simulink model "Appl_PaLearn_CtrlModel"  (R2018b)
settings: configuration reference "CodeConfig_10_ms" (kept outside this file)
undefined symbols (not defined in the file): CAL_LearnAllTimeMax_150s, CAL_LearnSingleTimeMax_60s, D_FirstMove, D_FourthlyMove, D_Invalid, D_SecondMove, D_ThirdlyMove, enDrAdjustEnable, FALSE, TRUE
libraries: DareLib x52, simulink x2
(part 1 of 2)
settings Model: Creator=Administrator  LastModifiedBy=Administrator
settings ConfigSetRef: SourceLocation=Base Workspace

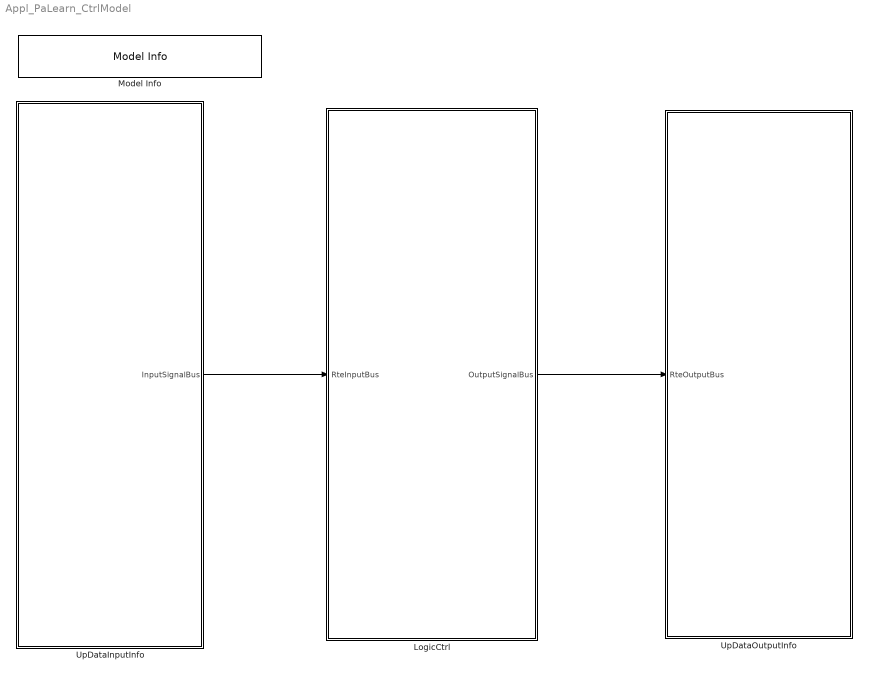
== system Appl_PaLearn_CtrlModel ==
  LogicCtrl : Subsystem  Priority=2  TreatAsAtomicUnit=on
      settings: RTWSystemCode=Nonreusable function  RTWFcnNameOpts=Use subsystem name
  Model Info : simulink/Model-Wide Utilities/Model Info  Frame=on  DisplayStringWithTags=Version：%<ModelVersion>  HorizontalTextAlignment=Center  LeftAlignmentValue=0.5
  UpDataInputInfo : Subsystem  Priority=1  TreatAsAtomicUnit=on
      settings: RTWSystemCode=Nonreusable function  RTWFcnNameOpts=Use subsystem name
  UpDataOutputInfo : Subsystem  Priority=3  TreatAsAtomicUnit=on
      settings: RTWSystemCode=Nonreusable function  RTWFcnNameOpts=Use subsystem name
  wires:
  LogicCtrl/1(OutputSignalBus) -> UpDataOutputInfo/1(RteOutputBus)
  UpDataInputInfo/1(InputSignalBus) -> LogicCtrl/1(RteInputBus)

== system Appl_PaLearn_CtrlModel/LogicCtrl ==
  RteInputBus : Inport
  LocalAdjustCtrl : Subsystem  Description=学习逻辑处理
      settings: AttributesFormatString=%<Description>
  OutputSignalBus : Outport
  wires:
  RteInputBus/1 -> LocalAdjustCtrl/1(RteInputBus)  "RteInputBus"
  LocalAdjustCtrl/1(OutputSignalBus) -> OutputSignalBus/1

== system Appl_PaLearn_CtrlModel/UpDataInputInfo ==
  InputSignalProcess : Subsystem  Description=数据处理
      settings: AttributesFormatString=%<Description>  RTWSystemCode=Nonreusable function  RTWFcnNameOpts=Use subsystem name
  RTE : Subsystem  Description=接口自动生成  TreatAsAtomicUnit=on
      settings: AttributesFormatString=%<Description>  RTWSystemCode=Nonreusable function  RTWFcnNameOpts=Use subsystem name
  InputSignalBus : Outport
  wires:
  InputSignalProcess/1(InputSignalBus) -> InputSignalBus/1
  RTE/1(RTE_Signal) -> InputSignalProcess/1(Rte_SignalBus)

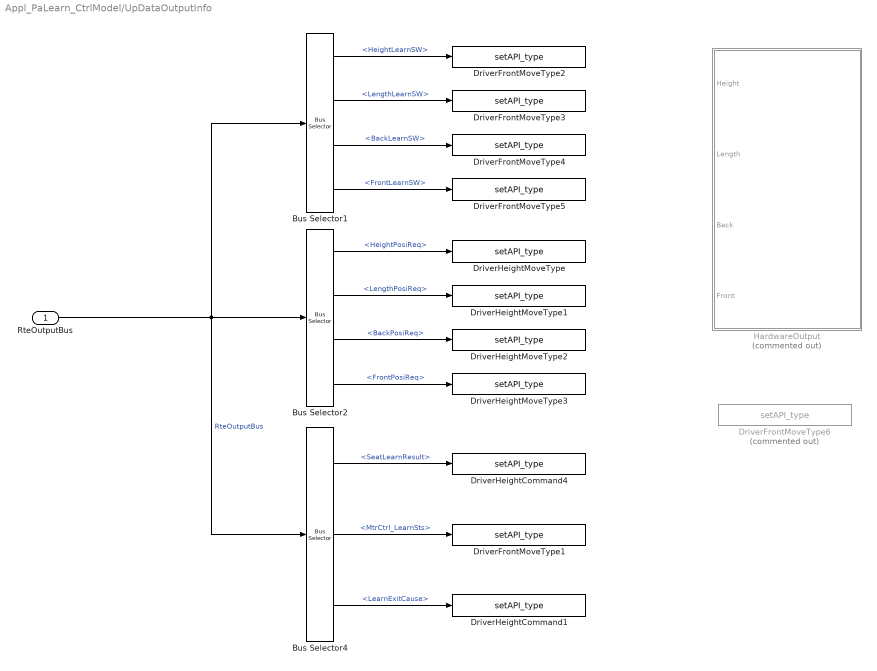
== system Appl_PaLearn_CtrlModel/UpDataOutputInfo ==
  RteOutputBus : Inport
  Bus Selector1 : BusSelector  OutputSignals=LearnOut.HeightLearnSW,LearnOut.LengthLearnSW,LearnOut.BackLearnSW,LearnOut.FrontLearnSW
  Bus Selector2 : BusSelector  OutputSignals=ResetOutBus.HeightPosiReq,ResetOutBus.LengthPosiReq,ResetOutBus.BackPosiReq,ResetOutBus.FrontPosiReq
  Bus Selector4 : BusSelector  OutputSignals=SeatLearnResult,LearnOut.MtrCtrl_LearnSts,LearnOut.LearnExitCause
  DriverFrontMoveType1 : DareLib/Dare/setAPI_type  g_funcname=Rte_SetVfb_PaLearnSts  g_param=""  g_type=uint8  g_enum=enLearnSts  g_size=-1
      settings: AttributesFormatString=%<g_funcname>  SourceProductName=Dare Library
  DriverFrontMoveType2 : DareLib/Dare/setAPI_type  g_funcname=Rte_SetVfb_PaHeightLearnCmd  g_param=""  g_type=uint8  g_enum=enSWMoveCmd  g_size=-1
      settings: AttributesFormatString=%<g_funcname>  SourceProductName=Dare Library
  DriverFrontMoveType3 : DareLib/Dare/setAPI_type  g_funcname=Rte_SetVfb_PaLengthLearnCmd  g_param=""  g_type=uint8  g_enum=enSWMoveCmd  g_size=-1
      settings: AttributesFormatString=%<g_funcname>  SourceProductName=Dare Library
  DriverFrontMoveType4 : DareLib/Dare/setAPI_type  g_funcname=Rte_SetVfb_PaBackLearnCmd  g_param=""  g_type=uint8  g_enum=enSWMoveCmd  g_size=-1
      settings: AttributesFormatString=%<g_funcname>  SourceProductName=Dare Library
  DriverFrontMoveType5 : DareLib/Dare/setAPI_type  g_funcname=Rte_SetVfb_PaFrontLearnCmd  g_param=""  g_type=uint8  g_enum=enSWMoveCmd  g_size=-1
      settings: AttributesFormatString=%<g_funcname>  SourceProductName=Dare Library
  DriverFrontMoveType6 : DareLib/Dare/setAPI_type  Commented=on  g_funcname=Rte_SetVfb_DrLearnResult  g_param=""  g_type=uint8  g_enum=enSeatAutoRunSts  g_size=-1
      settings: AttributesFormatString=%<g_funcname>  SourceProductName=Dare Library
  DriverHeightCommand1 : DareLib/Dare/setAPI_type  g_funcname=Rte_SetVfb_PaLearnExitCause  g_param=""  g_type=uint8  g_enum=enLearnExitCause  g_size=-1
      settings: AttributesFormatString=%<g_funcname>  SourceProductName=Dare Library
  DriverHeightCommand4 : DareLib/Dare/setAPI_type  g_funcname=Rte_SetVfb_PaLearnResult  g_param=""  g_type=uint8  g_size=-1
      settings: AttributesFormatString=%<g_funcname>  SourceProductName=Dare Library
  DriverHeightMoveType : DareLib/Dare/setAPI_type  g_funcname=Rte_SetVfb_PaHeightResetReqPosi  g_param=""  g_type=uint16  g_size=-1
      settings: AttributesFormatString=%<g_funcname>  SourceProductName=Dare Library
  DriverHeightMoveType1 : DareLib/Dare/setAPI_type  g_funcname=Rte_SetVfb_PaLengthResetReqPosi  g_param=""  g_type=uint16  g_size=-1
      settings: AttributesFormatString=%<g_funcname>  SourceProductName=Dare Library
  DriverHeightMoveType2 : DareLib/Dare/setAPI_type  g_funcname=Rte_SetVfb_PaBackResetReqPosi  g_param=""  g_type=uint16  g_size=-1
      settings: AttributesFormatString=%<g_funcname>  SourceProductName=Dare Library
  DriverHeightMoveType3 : DareLib/Dare/setAPI_type  g_funcname=Rte_SetVfb_PaFrontResetReqPosi  g_param=""  g_type=uint16  g_size=-1
      settings: AttributesFormatString=%<g_funcname>  SourceProductName=Dare Library
  HardwareOutput : Subsystem  Commented=on
  wires:
  RteOutputBus/1 -> Bus Selector4/1, Bus Selector1/1, Bus Selector2/1  "RteOutputBus"
  Bus Selector2/4 -> DriverHeightMoveType3/1  "<FrontPosiReq>"
  Bus Selector2/3 -> DriverHeightMoveType2/1  "<BackPosiReq>"
  Bus Selector2/2 -> DriverHeightMoveType1/1  "<LengthPosiReq>"
  Bus Selector2/1 -> DriverHeightMoveType/1  "<HeightPosiReq>"
  Bus Selector4/2 -> DriverFrontMoveType1/1  "<MtrCtrl_LearnSts>"
  Bus Selector4/1 -> DriverHeightCommand4/1  "<SeatLearnResult>"
  Bus Selector1/1 -> DriverFrontMoveType2/1  "<HeightLearnSW>"
  Bus Selector1/2 -> DriverFrontMoveType3/1  "<LengthLearnSW>"
  Bus Selector1/3 -> DriverFrontMoveType4/1  "<BackLearnSW>"
  Bus Selector1/4 -> DriverFrontMoveType5/1  "<FrontLearnSW>"
  Bus Selector4/3 -> DriverHeightCommand1/1  "<LearnExitCause>"

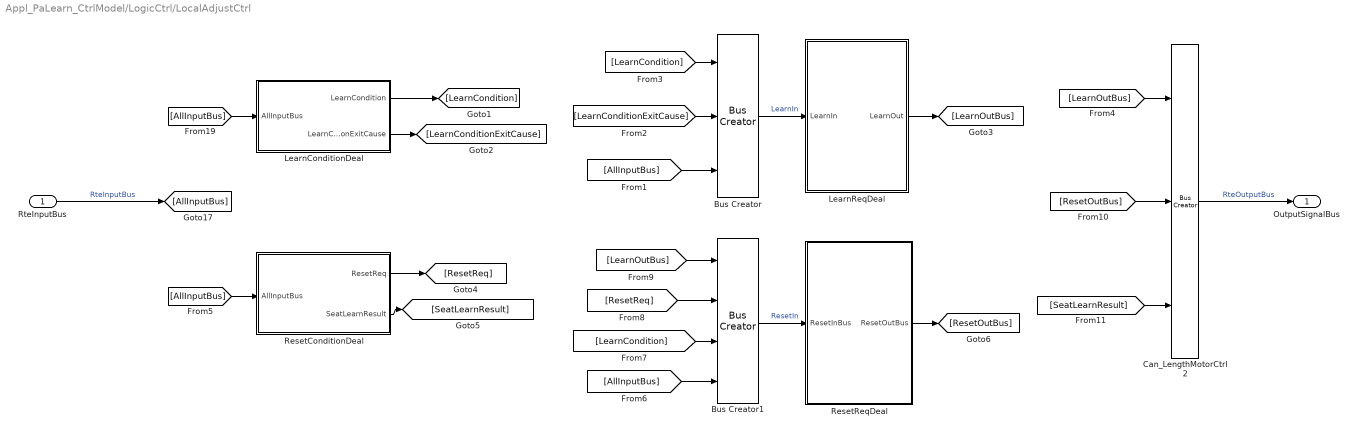
== system Appl_PaLearn_CtrlModel/LogicCtrl/LocalAdjustCtrl ==
  RteInputBus : Inport
  Bus Creator : BusCreator  Inputs=3
  Bus Creator1 : BusCreator  Inputs=4
  Can_LengthMotorCtrl2 : BusCreator  Inputs=3
  LearnConditionDeal : Subsystem
  LearnReqDeal : Subsystem
  ResetConditionDeal : Subsystem
  ResetReqDeal : Subsystem
  OutputSignalBus : Outport
  wires:
  RteInputBus/1 -> [AllInputBus]  "RteInputBus"
  [AllInputBus] -> Bus Creator/3
  [AllInputBus] -> LearnConditionDeal/1(AllInputBus)
  LearnConditionDeal/1(LearnCondition) -> [LearnCondition]
  LearnConditionDeal/2(LearnConditionExitCause) -> [LearnConditionExitCause]
  Bus Creator/1 -> LearnReqDeal/1(LearnIn)  "LearnIn"
  LearnReqDeal/1(LearnOut) -> [LearnOutBus]
  [LearnCondition] -> Bus Creator/1
  [LearnConditionExitCause] -> Bus Creator/2
  [LearnOutBus] -> Can_LengthMotorCtrl2/1
  Can_LengthMotorCtrl2/1 -> OutputSignalBus/1  "RteOutputBus"
  [LearnCondition] -> Bus Creator1/3
  [AllInputBus] -> Bus Creator1/4
  [ResetReq] -> Bus Creator1/2
  Bus Creator1/1 -> ResetReqDeal/1(ResetInBus)  "ResetIn"
  [LearnOutBus] -> Bus Creator1/1
  ResetReqDeal/1(ResetOutBus) -> [ResetOutBus]
  [ResetOutBus] -> Can_LengthMotorCtrl2/2
  [AllInputBus] -> ResetConditionDeal/1(AllInputBus)
  ResetConditionDeal/1(ResetReq) -> [ResetReq]
  ResetConditionDeal/2(SeatLearnResult) -> [SeatLearnResult]
  [SeatLearnResult] -> Can_LengthMotorCtrl2/3

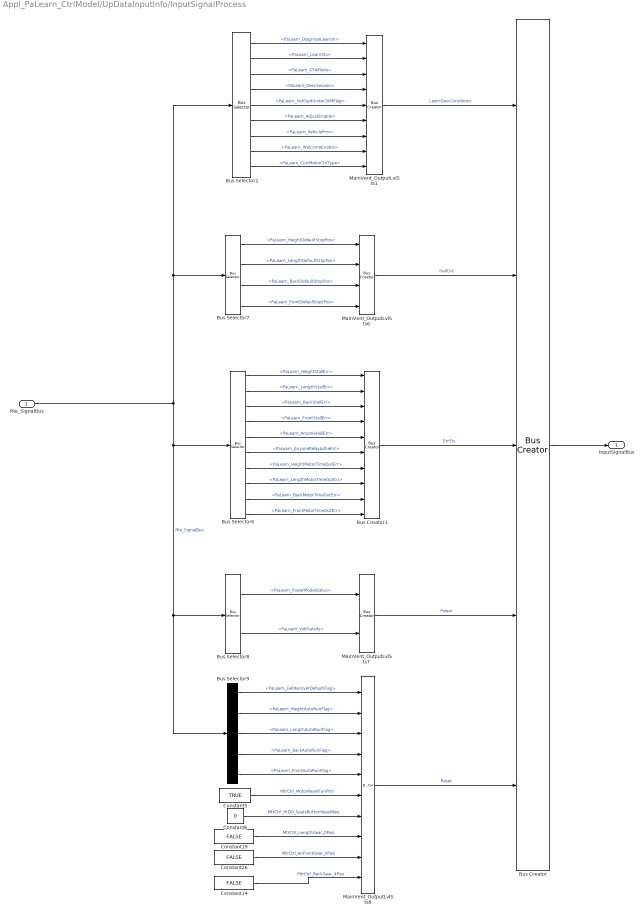
== system Appl_PaLearn_CtrlModel/UpDataInputInfo/InputSignalProcess ==
  Rte_SignalBus : Inport
  Bus Creator : BusCreator  Inputs=5
  Bus Creator1 : BusCreator  Inputs=10
  Bus Selector2 : BusSelector  OutputSignals=PaLearn_DiagnoseLearnIn,PaLearn_LearnSts,PaLearn_OTAMode,PaLearn_DescSession,PaLearn_VehSpdUnder3KMFlag,PaLearn_AdjustEnable,PaLearn_VehiclePrm,PaLearn_WelcomeEnable,PaLearn_CurrMotorCtrlType
  Bus Selector6 : BusSelector  OutputSignals=PaLearn_HeightStallErr,PaLearn_LengthStallErr,PaLearn_BackStallErr,PaLearn_FrontStallErr,PaLearn_AnyoneHallErr,PaLearn_AnyoneRelayAdheErr,PaLearn_HeightMotorTimeOutErr,PaLearn_LengthMotorTimeOutErr,PaLearn_BackMotorTimeOutErr,PaLearn_FrontMotorTimeOutErr
  Bus Selector7 : BusSelector  OutputSignals=PaLearn_HeightDefaultStopPos,PaLearn_LengthDefaultStopPos,PaLearn_BackDefaultStopPos,PaLearn_FrontDefaulStoptPos
  Bus Selector8 : BusSelector  OutputSignals=PaLearn_PowerModeStatus,PaLearn_VoltSatisfy
  Bus Selector9 : BusSelector  OutputSignals=PaLearn_GetRecoverDefaultFlag,PaLearn_HeightAutoRunFlag,PaLearn_LengthAutoRunFlag,PaLearn_BackAutoRunFlag,PaLearn_FrontAutoRunFlag
  Constant14 : Constant  Value=FALSE
  Constant19 : Constant  Value=FALSE
  Constant26 : Constant  Value=FALSE
  Constant5 : Constant  Value=TRUE
  Constant6 : Constant  Value=0
  MainVent_OutputLvlSts1 : BusCreator  Inputs=9
  MainVent_OutputLvlSts6 : BusCreator  Inputs=4
  MainVent_OutputLvlSts7 : BusCreator  Inputs=2
  MainVent_OutputLvlSts8 : BusCreator  Inputs=10
  InputSignalBus : Outport
  wires:
  Bus Creator/1 -> InputSignalBus/1
  Rte_SignalBus/1 -> Bus Selector2/1, Bus Selector7/1, Bus Selector9/1, Bus Selector8/1, Bus Selector6/1  "Rte_SignalBus"
  MainVent_OutputLvlSts7/1 -> Bus Creator/4  "Power"
  Bus Creator1/1 -> Bus Creator/3  "ErrSts"
  MainVent_OutputLvlSts1/1 -> Bus Creator/1  "LearnDescConditions"
  MainVent_OutputLvlSts6/1 -> Bus Creator/2  "HallCnt"
  MainVent_OutputLvlSts8/1 -> Bus Creator/5  "Reset"
  Bus Selector9/1 -> MainVent_OutputLvlSts8/1  "<PaLearn_GetRecoverDefaultFlag>"
  Bus Selector9/2 -> MainVent_OutputLvlSts8/2  "<PaLearn_HeightAutoRunFlag>"
  Bus Selector9/3 -> MainVent_OutputLvlSts8/3  "<PaLearn_LengthAutoRunFlag>"
  Bus Selector9/4 -> MainVent_OutputLvlSts8/4  "<PaLearn_BackAutoRunFlag>"
  Bus Selector9/5 -> MainVent_OutputLvlSts8/5  "<PaLearn_FrontAutoRunFlag>"
  Constant19/1 -> MainVent_OutputLvlSts8/8  "MtrCtrl_LengthGear_0Posi"
  Constant5/1 -> MainVent_OutputLvlSts8/6  "MtrCtrl_MotorResetFunPrm"
  Constant6/1 -> MainVent_OutputLvlSts8/7  "MtrCtrl_HIDO_SeatsButtonResetReq"
  Constant26/1 -> MainVent_OutputLvlSts8/9  "MtrCtrl_enFrontGear_0Posi"
  Constant14/1 -> MainVent_OutputLvlSts8/10  "MtrCtrl_BackGear_4Posi"
  Bus Selector7/3 -> MainVent_OutputLvlSts6/3  "<PaLearn_BackDefaultStopPos>"
  Bus Selector7/2 -> MainVent_OutputLvlSts6/2  "<PaLearn_LengthDefaultStopPos>"
  Bus Selector7/4 -> MainVent_OutputLvlSts6/4  "<PaLearn_FrontDefaulStoptPos>"
  Bus Selector7/1 -> MainVent_OutputLvlSts6/1  "<PaLearn_HeightDefaultStopPos>"
  Bus Selector6/1 -> Bus Creator1/1  "<PaLearn_HeightStallErr>"
  Bus Selector6/2 -> Bus Creator1/2  "<PaLearn_LengthStallErr>"
  Bus Selector6/3 -> Bus Creator1/3  "<PaLearn_BackStallErr>"
  Bus Selector6/4 -> Bus Creator1/4  "<PaLearn_FrontStallErr>"
  Bus Selector6/5 -> Bus Creator1/5  "<PaLearn_AnyoneHallErr>"
  Bus Selector6/6 -> Bus Creator1/6  "<PaLearn_AnyoneRelayAdheErr>"
  Bus Selector6/7 -> Bus Creator1/7  "<PaLearn_HeightMotorTimeOutErr>"
  Bus Selector6/8 -> Bus Creator1/8  "<PaLearn_LengthMotorTimeOutErr>"
  Bus Selector6/9 -> Bus Creator1/9  "<PaLearn_BackMotorTimeOutErr>"
  Bus Selector6/10 -> Bus Creator1/10  "<PaLearn_FrontMotorTimeOutErr>"
  Bus Selector8/2 -> MainVent_OutputLvlSts7/2  "<PaLearn_VoltSatisfy>"
  Bus Selector8/1 -> MainVent_OutputLvlSts7/1  "<PaLearn_PowerModeStatus>"
  Bus Selector2/1 -> MainVent_OutputLvlSts1/1  "<PaLearn_DiagnoseLearnIn>"
  Bus Selector2/2 -> MainVent_OutputLvlSts1/2  "<PaLearn_LearnSts>"
  Bus Selector2/3 -> MainVent_OutputLvlSts1/3  "<PaLearn_OTAMode>"
  Bus Selector2/4 -> MainVent_OutputLvlSts1/4  "<PaLearn_DescSession>"
  Bus Selector2/5 -> MainVent_OutputLvlSts1/5  "<PaLearn_VehSpdUnder3KMFlag>"
  Bus Selector2/6 -> MainVent_OutputLvlSts1/6  "<PaLearn_AdjustEnable>"
  Bus Selector2/7 -> MainVent_OutputLvlSts1/7  "<PaLearn_VehiclePrm>"
  Bus Selector2/8 -> MainVent_OutputLvlSts1/8  "<PaLearn_WelcomeEnable>"
  Bus Selector2/9 -> MainVent_OutputLvlSts1/9  "<PaLearn_CurrMotorCtrlType>"

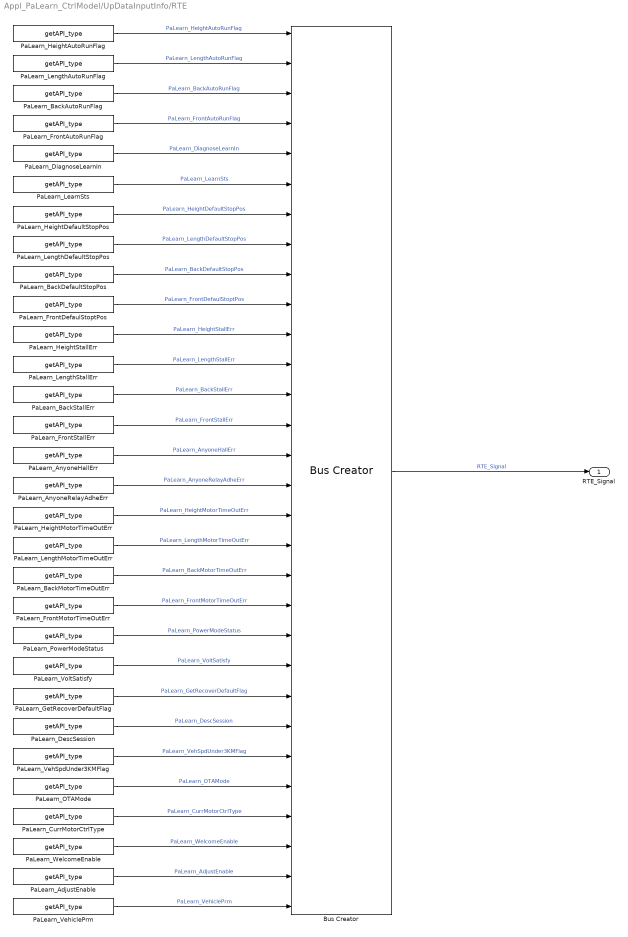
== system Appl_PaLearn_CtrlModel/UpDataInputInfo/RTE ==
  Bus Creator : BusCreator  Inputs=30
  PaLearn_AdjustEnable : DareLib/Dare/getAPI_type  g_funcname=Srvl_GetMemIndexDataU8  g_param=EN_MemIndex_PaAdjustConfig  g_type=uint8  g_size=-1
      settings: AttributesFormatString=%<g_funcname>  SourceProductName=Dare Library
  PaLearn_AnyoneHallErr : DareLib/Dare/getAPI_type  g_funcname=Rte_GetVfb_PaAnyoneHallErr  g_param=""  g_type=uint8  g_size=-1
      settings: AttributesFormatString=%<g_funcname>  SourceProductName=Dare Library
  PaLearn_AnyoneRelayAdheErr : DareLib/Dare/getAPI_type  g_funcname=Rte_GetVfb_PaAnyoneRelayAdheErr  g_param=""  g_type=uint8  g_size=-1
      settings: AttributesFormatString=%<g_funcname>  SourceProductName=Dare Library
  PaLearn_BackAutoRunFlag : DareLib/Dare/getAPI_type  g_funcname=Rte_GetVfb_PaBackAutoRunFlag  g_param=""  g_type=uint8  g_enum=enSeatAutoRunSts  g_size=-1
      settings: AttributesFormatString=%<g_funcname>  SourceProductName=Dare Library
  PaLearn_BackDefaultStopPos : DareLib/Dare/getAPI_type  g_funcname=Cdd_GetMotorHardStop  g_param=EN_PassengerBack  g_type=uint16  g_size=-1
      settings: AttributesFormatString=%<g_funcname>  SourceProductName=Dare Library
  PaLearn_BackMotorTimeOutErr : DareLib/Dare/getAPI_type  g_funcname=Rte_GetVfb_PaBackMotorTimeOutErr  g_param=""  g_type=uint8  g_size=-1
      settings: AttributesFormatString=%<g_funcname>  SourceProductName=Dare Library
  PaLearn_BackStallErr : DareLib/Dare/getAPI_type  g_funcname=Rte_GetVfb_PaBackStallErr  g_param=""  g_type=uint8  g_size=-1
      settings: AttributesFormatString=%<g_funcname>  SourceProductName=Dare Library
  PaLearn_CurrMotorCtrlType : DareLib/Dare/getAPI_type  g_funcname=Rte_GetVfb_PaMoveType  g_param=""  g_type=uint8  g_enum=enSeatMotorRunTye  g_size=-1
      settings: AttributesFormatString=%<g_funcname>  SourceProductName=Dare Library
  PaLearn_DescSession : DareLib/Dare/getAPI_type  g_funcname=DescGetcDescSession  g_param=""  g_type=uint8  g_size=-1
      settings: AttributesFormatString=%<g_funcname>  SourceProductName=Dare Library
  PaLearn_DiagnoseLearnIn : DareLib/Dare/getAPI_type  g_funcname=Rte_GetVfb_PaLearnEnable  g_param=""  g_type=uint8  g_size=-1
      settings: AttributesFormatString=%<g_funcname>  SourceProductName=Dare Library
  PaLearn_FrontAutoRunFlag : DareLib/Dare/getAPI_type  g_funcname=Rte_GetVfb_PaFrontAutoRunFlag  g_param=""  g_type=uint8  g_enum=enSeatAutoRunSts  g_size=-1
      settings: AttributesFormatString=%<g_funcname>  SourceProductName=Dare Library
  PaLearn_FrontDefaulStoptPos : DareLib/Dare/getAPI_type  g_funcname=Cdd_GetMotorHardStop  g_param=EN_PaResever_2  g_type=uint16  g_size=-1
      settings: AttributesFormatString=%<g_funcname>  SourceProductName=Dare Library
  PaLearn_FrontMotorTimeOutErr : DareLib/Dare/getAPI_type  g_funcname=Rte_GetVfb_PaFrontMotorTimeOutErr  g_param=""  g_type=uint8  g_size=-1
      settings: AttributesFormatString=%<g_funcname>  SourceProductName=Dare Library
  PaLearn_FrontStallErr : DareLib/Dare/getAPI_type  g_funcname=Rte_GetVfb_PaFrontStallErr  g_param=""  g_type=uint8  g_size=-1
      settings: AttributesFormatString=%<g_funcname>  SourceProductName=Dare Library
  PaLearn_GetRecoverDefaultFlag : DareLib/Dare/getAPI_type  g_funcname=GetRecoverDefaultFlag  g_param=""  g_type=uint8  g_size=-1
      settings: AttributesFormatString=%<g_funcname>  SourceProductName=Dare Library
  PaLearn_HeightAutoRunFlag : DareLib/Dare/getAPI_type  g_funcname=Rte_GetVfb_PaHeightAutoRunFlag  g_param=""  g_type=uint8  g_enum=enSeatAutoRunSts  g_size=-1
      settings: AttributesFormatString=%<g_funcname>  SourceProductName=Dare Library
  PaLearn_HeightDefaultStopPos : DareLib/Dare/getAPI_type  g_funcname=Cdd_GetMotorHardStop  g_param=EN_PaResever_1  g_type=uint16  g_size=-1
      settings: AttributesFormatString=%<g_funcname>  SourceProductName=Dare Library
  PaLearn_HeightMotorTimeOutErr : DareLib/Dare/getAPI_type  g_funcname=Rte_GetVfb_PaHeightMotorTimeOutErr  g_param=""  g_type=uint8  g_size=-1
      settings: AttributesFormatString=%<g_funcname>  SourceProductName=Dare Library
  PaLearn_HeightStallErr : DareLib/Dare/getAPI_type  g_funcname=Rte_GetVfb_PaHeightStallErr  g_param=""  g_type=uint8  g_size=-1
      settings: AttributesFormatString=%<g_funcname>  SourceProductName=Dare Library
  PaLearn_LearnSts : DareLib/Dare/getAPI_type  g_funcname=Rte_GetVfb_PaLearnSts  g_param=""  g_type=uint8  g_size=-1
      settings: AttributesFormatString=%<g_funcname>  SourceProductName=Dare Library
  PaLearn_LengthAutoRunFlag : DareLib/Dare/getAPI_type  g_funcname=Rte_GetVfb_PaLengthAutoRunFlag  g_param=""  g_type=uint8  g_enum=enSeatAutoRunSts  g_size=-1
      settings: AttributesFormatString=%<g_funcname>  SourceProductName=Dare Library
  PaLearn_LengthDefaultStopPos : DareLib/Dare/getAPI_type  g_funcname=Cdd_GetMotorHardStop  g_param=EN_PassengerLength  g_type=uint16  g_size=-1
      settings: AttributesFormatString=%<g_funcname>  SourceProductName=Dare Library
  PaLearn_LengthMotorTimeOutErr : DareLib/Dare/getAPI_type  g_funcname=Rte_GetVfb_PaLengthMotorTimeOutErr  g_param=""  g_type=uint8  g_size=-1
      settings: AttributesFormatString=%<g_funcname>  SourceProductName=Dare Library
  PaLearn_LengthStallErr : DareLib/Dare/getAPI_type  g_funcname=Rte_GetVfb_PaLengthStallErr  g_param=""  g_type=uint8  g_size=-1
      settings: AttributesFormatString=%<g_funcname>  SourceProductName=Dare Library
  PaLearn_OTAMode : DareLib/Dare/getAPI_type  g_funcname=Vfb_Reserved_0  g_param=""  g_type=uint8  g_size=-1
      settings: AttributesFormatString=%<g_funcname>  SourceProductName=Dare Library
  PaLearn_PowerModeStatus : DareLib/Dare/getAPI_type  g_funcname=Rte_GetVfb_PowerMode  g_param=""  g_type=uint8  g_enum=enIgnSts  g_size=-1
      settings: AttributesFormatString=%<g_funcname>  SourceProductName=Dare Library
  PaLearn_VehSpdUnder3KMFlag : DareLib/Dare/getAPI_type  g_funcname=DescCheckVehSpd  g_param=""  g_type=uint8  g_size=-1
      settings: AttributesFormatString=%<g_funcname>  SourceProductName=Dare Library
  PaLearn_VehiclePrm : DareLib/Dare/getAPI_type  g_funcname=Srvl_GetMemIndexDataU8  g_param=EN_MemIndex_Heat_CarType  g_type=uint8  g_enum=enVehTypePrm  g_size=-1
      settings: AttributesFormatString=%<g_funcname>  SourceProductName=Dare Library
  PaLearn_VoltSatisfy : DareLib/Dare/getAPI_type  g_funcname=Rte_GetVfb_VoltSatisfy  g_param=""  g_type=uint8  g_size=-1
      settings: AttributesFormatString=%<g_funcname>  SourceProductName=Dare Library
  PaLearn_WelcomeEnable : DareLib/Dare/getAPI_type  g_funcname=Srvl_GetMemIndexDataU8  g_param=EN_MemIndex_PaMemoryConfig  g_type=uint8  g_size=-1
      settings: AttributesFormatString=%<g_funcname>  SourceProductName=Dare Library
  RTE_Signal : Outport
  wires:
  Bus Creator/1 -> RTE_Signal/1  "RTE_Signal"
  PaLearn_HeightAutoRunFlag/1 -> Bus Creator/1  "PaLearn_HeightAutoRunFlag"
  PaLearn_LengthAutoRunFlag/1 -> Bus Creator/2  "PaLearn_LengthAutoRunFlag"
  PaLearn_BackAutoRunFlag/1 -> Bus Creator/3  "PaLearn_BackAutoRunFlag"
  PaLearn_FrontAutoRunFlag/1 -> Bus Creator/4  "PaLearn_FrontAutoRunFlag"
  PaLearn_DiagnoseLearnIn/1 -> Bus Creator/5  "PaLearn_DiagnoseLearnIn"
  PaLearn_LearnSts/1 -> Bus Creator/6  "PaLearn_LearnSts"
  PaLearn_HeightDefaultStopPos/1 -> Bus Creator/7  "PaLearn_HeightDefaultStopPos"
  PaLearn_LengthDefaultStopPos/1 -> Bus Creator/8  "PaLearn_LengthDefaultStopPos"
  PaLearn_BackDefaultStopPos/1 -> Bus Creator/9  "PaLearn_BackDefaultStopPos"
  PaLearn_FrontDefaulStoptPos/1 -> Bus Creator/10  "PaLearn_FrontDefaulStoptPos"
  PaLearn_HeightStallErr/1 -> Bus Creator/11  "PaLearn_HeightStallErr"
  PaLearn_LengthStallErr/1 -> Bus Creator/12  "PaLearn_LengthStallErr"
  PaLearn_BackStallErr/1 -> Bus Creator/13  "PaLearn_BackStallErr"
  PaLearn_FrontStallErr/1 -> Bus Creator/14  "PaLearn_FrontStallErr"
  PaLearn_AnyoneHallErr/1 -> Bus Creator/15  "PaLearn_AnyoneHallErr"
  PaLearn_AnyoneRelayAdheErr/1 -> Bus Creator/16  "PaLearn_AnyoneRelayAdheErr"
  PaLearn_HeightMotorTimeOutErr/1 -> Bus Creator/17  "PaLearn_HeightMotorTimeOutErr"
  PaLearn_LengthMotorTimeOutErr/1 -> Bus Creator/18  "PaLearn_LengthMotorTimeOutErr"
  PaLearn_BackMotorTimeOutErr/1 -> Bus Creator/19  "PaLearn_BackMotorTimeOutErr"
  PaLearn_FrontMotorTimeOutErr/1 -> Bus Creator/20  "PaLearn_FrontMotorTimeOutErr"
  PaLearn_PowerModeStatus/1 -> Bus Creator/21  "PaLearn_PowerModeStatus"
  PaLearn_VoltSatisfy/1 -> Bus Creator/22  "PaLearn_VoltSatisfy"
  PaLearn_GetRecoverDefaultFlag/1 -> Bus Creator/23  "PaLearn_GetRecoverDefaultFlag"
  PaLearn_DescSession/1 -> Bus Creator/24  "PaLearn_DescSession"
  PaLearn_VehSpdUnder3KMFlag/1 -> Bus Creator/25  "PaLearn_VehSpdUnder3KMFlag"
  PaLearn_OTAMode/1 -> Bus Creator/26  "PaLearn_OTAMode"
  PaLearn_CurrMotorCtrlType/1 -> Bus Creator/27  "PaLearn_CurrMotorCtrlType"
  PaLearn_WelcomeEnable/1 -> Bus Creator/28  "PaLearn_WelcomeEnable"
  PaLearn_AdjustEnable/1 -> Bus Creator/29  "PaLearn_AdjustEnable"
  PaLearn_VehiclePrm/1 -> Bus Creator/30  "PaLearn_VehiclePrm"

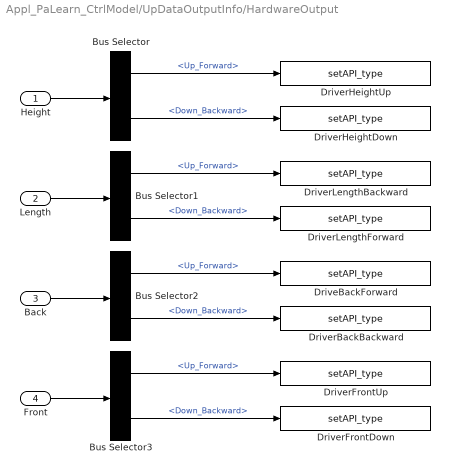
== system Appl_PaLearn_CtrlModel/UpDataOutputInfo/HardwareOutput ==
  Height : Inport
  Length : Inport  Port=2
  Back : Inport  Port=3
  Front : Inport  Port=4
  Bus Selector{,1..3} (4 alike) : BusSelector  OutputSignals=Up_Forward,Down_Backward
  DriveBackForward : DareLib/Dare/setAPI_type  g_funcname=Ecual_GpioWriteCh  g_param=EN_MCU_PIN6_RELAY_DRV  g_type=uint8  g_size=-1
      settings: AttributesFormatString=%<g_funcname>  SourceProductName=Dare Library
  DriverBackBackward : DareLib/Dare/setAPI_type  g_funcname=Ecual_GpioWriteCh  g_param=EN_MCU_PIN7_RELAY_DRV  g_type=uint8  g_size=-1
      settings: AttributesFormatString=%<g_funcname>  SourceProductName=Dare Library
  DriverFrontDown : DareLib/Dare/setAPI_type  g_funcname=Ecual_GpioWriteCh  g_param=EN_MCU_PIN4_RELAY_DRV  g_type=uint8  g_size=-1
      settings: AttributesFormatString=%<g_funcname>  SourceProductName=Dare Library
  DriverFrontUp : DareLib/Dare/setAPI_type  g_funcname=Ecual_GpioWriteCh  g_param=EN_MCU_PIN9_RELAY_DRV  g_type=uint8  g_size=-1
      settings: AttributesFormatString=%<g_funcname>  SourceProductName=Dare Library
  DriverHeightDown : DareLib/Dare/setAPI_type  g_funcname=Ecual_GpioWriteCh  g_param=EN_MCU_PIN1_RELAY_DRV  g_type=uint8  g_size=-1
      settings: AttributesFormatString=%<g_funcname>  SourceProductName=Dare Library
  DriverHeightUp : DareLib/Dare/setAPI_type  g_funcname=Ecual_GpioWriteCh  g_param=EN_MCU_PIN2_RELAY_DRV  g_type=uint8  g_size=-1
      settings: AttributesFormatString=%<g_funcname>  SourceProductName=Dare Library
  DriverLengthBackward : DareLib/Dare/setAPI_type  g_funcname=Ecual_GpioWriteCh  g_param=EN_MCU_PIN8_RELAY_DRV  g_type=uint8  g_size=-1
      settings: AttributesFormatString=%<g_funcname>  SourceProductName=Dare Library
  DriverLengthForward : DareLib/Dare/setAPI_type  g_funcname=Ecual_GpioWriteCh  g_param=EN_MCU_PIN3_RELAY_DRV  g_type=uint8  g_size=-1
      settings: AttributesFormatString=%<g_funcname>  SourceProductName=Dare Library
  wires:
  Height/1 -> Bus Selector/1
  Bus Selector/1 -> DriverHeightUp/1  "<Up_Forward>"
  Bus Selector/2 -> DriverHeightDown/1  "<Down_Backward>"
  Length/1 -> Bus Selector1/1
  Bus Selector1/1 -> DriverLengthBackward/1  "<Up_Forward>"
  Bus Selector1/2 -> DriverLengthForward/1  "<Down_Backward>"
  Back/1 -> Bus Selector2/1
  Bus Selector2/1 -> DriveBackForward/1  "<Up_Forward>"
  Bus Selector2/2 -> DriverBackBackward/1  "<Down_Backward>"
  Front/1 -> Bus Selector3/1
  Bus Selector3/1 -> DriverFrontUp/1  "<Up_Forward>"
  Bus Selector3/2 -> DriverFrontDown/1  "<Down_Backward>"

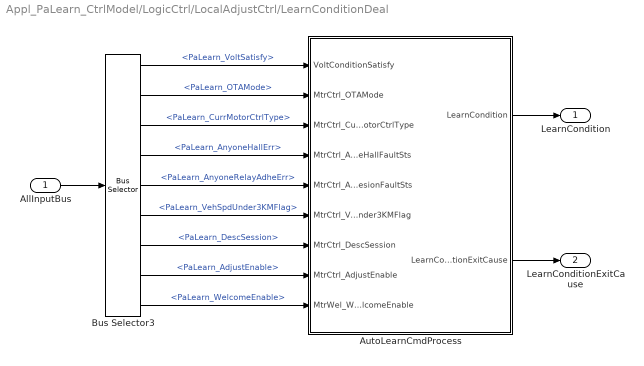
== system Appl_PaLearn_CtrlModel/LogicCtrl/LocalAdjustCtrl/LearnConditionDeal ==
  AllInputBus : Inport
  AutoLearnCmdProcess : Stateflow chart  TreatAsAtomicUnit=on
  Bus Selector3 : BusSelector  OutputSignals=Power.PaLearn_VoltSatisfy,LearnDescConditions.PaLearn_OTAMode,LearnDescConditions.PaLearn_CurrMotorCtrlType,ErrSts.PaLearn_AnyoneHallErr,ErrSts.PaLearn_AnyoneRelayAdheErr,LearnDescConditions.PaLearn_VehSpdUnder3KMFlag,LearnDescConditions.PaLearn_DescSession,LearnDescConditions.PaLearn_AdjustEnable,LearnDescConditions.PaLearn_WelcomeEnable
  LearnCondition : Outport
  LearnConditionExitCause : Outport  Port=2
  wires:
  Bus Selector3/9 -> AutoLearnCmdProcess/9(MtrWel_WelcomeEnable)  "<PaLearn_WelcomeEnable>"
  Bus Selector3/1 -> AutoLearnCmdProcess/1(VoltConditionSatisfy)  "<PaLearn_VoltSatisfy>"
  Bus Selector3/2 -> AutoLearnCmdProcess/2(MtrCtrl_OTAMode)  "<PaLearn_OTAMode>"
  Bus Selector3/4 -> AutoLearnCmdProcess/4(MtrCtrl_AnyoneHallFaultSts)  "<PaLearn_AnyoneHallErr>"
  Bus Selector3/8 -> AutoLearnCmdProcess/8(MtrCtrl_AdjustEnable)  "<PaLearn_AdjustEnable>"
  Bus Selector3/3 -> AutoLearnCmdProcess/3(MtrCtrl_CurrMotorCtrlType)  "<PaLearn_CurrMotorCtrlType>"
  Bus Selector3/5 -> AutoLearnCmdProcess/5(MtrCtrl_AnyoneAdhesionFaultSts)  "<PaLearn_AnyoneRelayAdheErr>"
  Bus Selector3/6 -> AutoLearnCmdProcess/6(MtrCtrl_VehSpdUnder3KMFlag)  "<PaLearn_VehSpdUnder3KMFlag>"
  Bus Selector3/7 -> AutoLearnCmdProcess/7(MtrCtrl_DescSession)  "<PaLearn_DescSession>"
  AutoLearnCmdProcess/2(LearnConditionExitCause) -> LearnConditionExitCause/1
  AutoLearnCmdProcess/1(LearnCondition) -> LearnCondition/1
  AllInputBus/1 -> Bus Selector3/1

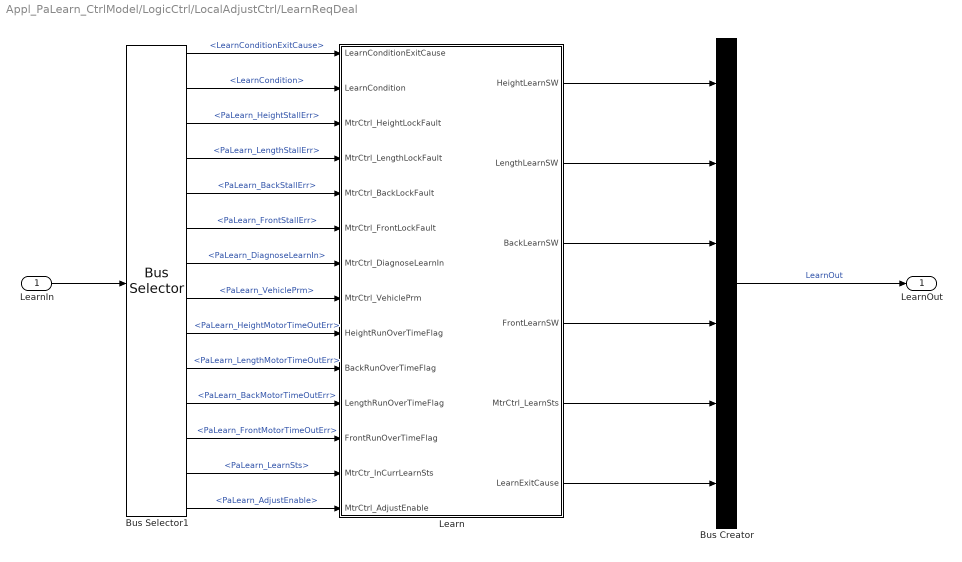
== system Appl_PaLearn_CtrlModel/LogicCtrl/LocalAdjustCtrl/LearnReqDeal ==
  LearnIn : Inport
  Bus Creator : BusCreator  Inputs=6
  Bus Selector1 : BusSelector  OutputSignals=LearnConditionExitCause,LearnCondition,RteInputBus.ErrSts.PaLearn_HeightStallErr,RteInputBus.ErrSts.PaLearn_LengthStallErr,RteInputBus.ErrSts.PaLearn_BackStallErr,RteInputBus.ErrSts.PaLearn_FrontStallErr,RteInputBus.LearnDescConditions.PaLearn_DiagnoseLearnIn,RteInputBus.LearnDescConditions.PaLearn_VehiclePrm,RteInputBus.ErrSts.PaLearn_HeightMotorTimeOutErr,RteInputBus.ErrSts.PaLearn_LengthMotorTimeOutErr,RteInputBus.ErrSts.PaLearn_BackMotorTimeOutErr,RteInputBus.ErrSts.PaLearn_FrontMotorTimeOutErr,RteInputBus.LearnDescConditions.PaLearn_LearnSts,RteInputBus.LearnDescConditions.PaLearn_AdjustEnable
  Learn : Stateflow chart  TreatAsAtomicUnit=on
  LearnOut : Outport
  wires:
  Bus Selector1/7 -> Learn/7(MtrCtrl_DiagnoseLearnIn)  "<PaLearn_DiagnoseLearnIn>"
  Bus Selector1/8 -> Learn/8(MtrCtrl_VehiclePrm)  "<PaLearn_VehiclePrm>"
  Bus Selector1/10 -> Learn/10(BackRunOverTimeFlag)  "<PaLearn_LengthMotorTimeOutErr>"
  Bus Selector1/3 -> Learn/3(MtrCtrl_HeightLockFault)  "<PaLearn_HeightStallErr>"
  Bus Selector1/5 -> Learn/5(MtrCtrl_BackLockFault)  "<PaLearn_BackStallErr>"
  Bus Selector1/13 -> Learn/13(MtrCtr_InCurrLearnSts)  "<PaLearn_LearnSts>"
  Bus Selector1/4 -> Learn/4(MtrCtrl_LengthLockFault)  "<PaLearn_LengthStallErr>"
  Bus Selector1/14 -> Learn/14(MtrCtrl_AdjustEnable)  "<PaLearn_AdjustEnable>"
  Bus Selector1/6 -> Learn/6(MtrCtrl_FrontLockFault)  "<PaLearn_FrontStallErr>"
  Bus Selector1/11 -> Learn/11(LengthRunOverTimeFlag)  "<PaLearn_BackMotorTimeOutErr>"
  Bus Selector1/12 -> Learn/12(FrontRunOverTimeFlag)  "<PaLearn_FrontMotorTimeOutErr>"
  Bus Selector1/9 -> Learn/9(HeightRunOverTimeFlag)  "<PaLearn_HeightMotorTimeOutErr>"
  LearnIn/1 -> Bus Selector1/1
  Bus Creator/1 -> LearnOut/1  "LearnOut"
  Learn/3(BackLearnSW) -> Bus Creator/3
  Learn/2(LengthLearnSW) -> Bus Creator/2
  Learn/4(FrontLearnSW) -> Bus Creator/4
  Learn/1(HeightLearnSW) -> Bus Creator/1
  Learn/5(MtrCtrl_LearnSts) -> Bus Creator/5
  Learn/6(LearnExitCause) -> Bus Creator/6
  Bus Selector1/2 -> Learn/2(LearnCondition)  "<LearnCondition>"
  Bus Selector1/1 -> Learn/1(LearnConditionExitCause)  "<LearnConditionExitCause>"

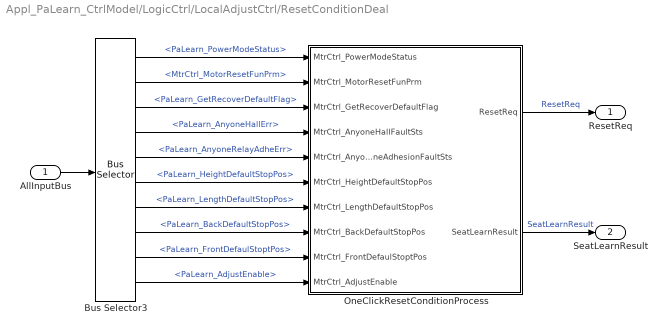
== system Appl_PaLearn_CtrlModel/LogicCtrl/LocalAdjustCtrl/ResetConditionDeal ==
  AllInputBus : Inport
  Bus Selector3 : BusSelector  OutputSignals=Power.PaLearn_PowerModeStatus,Reset.MtrCtrl_MotorResetFunPrm,Reset.PaLearn_GetRecoverDefaultFlag,ErrSts.PaLearn_AnyoneHallErr,ErrSts.PaLearn_AnyoneRelayAdheErr,HallCnt.PaLearn_HeightDefaultStopPos,HallCnt.PaLearn_LengthDefaultStopPos,HallCnt.PaLearn_BackDefaultStopPos,HallCnt.PaLearn_FrontDefaulStoptPos,LearnDescConditions.PaLearn_AdjustEnable
  OneClickResetConditionProcess : Subsystem  Description=一键复位条件处理（BM400）
  ResetReq : Outport
  SeatLearnResult : Outport  Port=2
  wires:
  Bus Selector3/4 -> OneClickResetConditionProcess/4(MtrCtrl_AnyoneHallFaultSts)  "<PaLearn_AnyoneHallErr>"
  Bus Selector3/2 -> OneClickResetConditionProcess/2(MtrCtrl_MotorResetFunPrm)  "<MtrCtrl_MotorResetFunPrm>"
  Bus Selector3/10 -> OneClickResetConditionProcess/10(MtrCtrl_AdjustEnable)  "<PaLearn_AdjustEnable>"
  Bus Selector3/3 -> OneClickResetConditionProcess/3(MtrCtrl_GetRecoverDefaultFlag)  "<PaLearn_GetRecoverDefaultFlag>"
  Bus Selector3/8 -> OneClickResetConditionProcess/8(MtrCtrl_BackDefaultStopPos)  "<PaLearn_BackDefaultStopPos>"
  Bus Selector3/1 -> OneClickResetConditionProcess/1(MtrCtrl_PowerModeStatus)  "<PaLearn_PowerModeStatus>"
  Bus Selector3/5 -> OneClickResetConditionProcess/5(MtrCtrl_AnyoneAdhesionFaultSts)  "<PaLearn_AnyoneRelayAdheErr>"
  Bus Selector3/6 -> OneClickResetConditionProcess/6(MtrCtrl_HeightDefaultStopPos)  "<PaLearn_HeightDefaultStopPos>"
  Bus Selector3/7 -> OneClickResetConditionProcess/7(MtrCtrl_LengthDefaultStopPos)  "<PaLearn_LengthDefaultStopPos>"
  Bus Selector3/9 -> OneClickResetConditionProcess/9(MtrCtrl_FrontDefaulStoptPos)  "<PaLearn_FrontDefaulStoptPos>"
  OneClickResetConditionProcess/2(SeatLearnResult) -> SeatLearnResult/1  "SeatLearnResult"
  AllInputBus/1 -> Bus Selector3/1
  OneClickResetConditionProcess/1(ResetReq) -> ResetReq/1  "ResetReq"

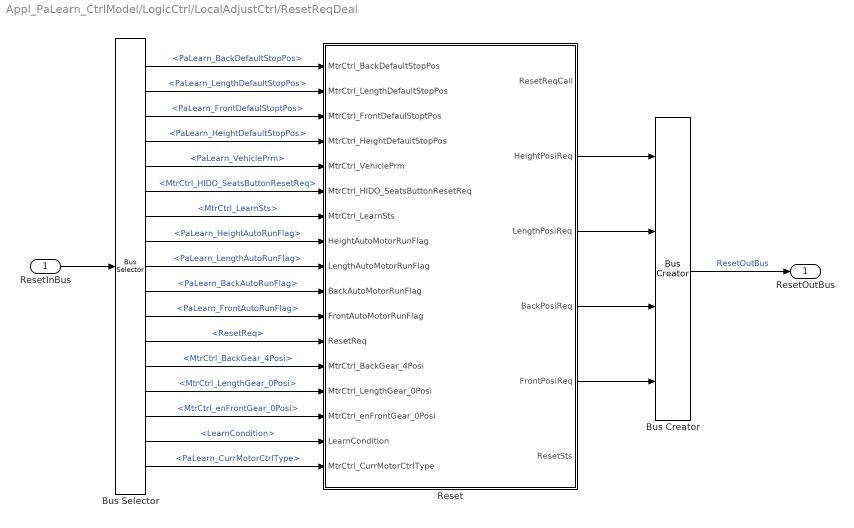
== system Appl_PaLearn_CtrlModel/LogicCtrl/LocalAdjustCtrl/ResetReqDeal ==
  ResetInBus : Inport
  Bus Creator : BusCreator  Inputs=4
  Bus Selector : BusSelector  OutputSignals=RteInputBus.HallCnt.PaLearn_BackDefaultStopPos,RteInputBus.HallCnt.PaLearn_LengthDefaultStopPos,RteInputBus.HallCnt.PaLearn_FrontDefaulStoptPos,RteInputBus.HallCnt.PaLearn_HeightDefaultStopPos,RteInputBus.LearnDescConditions.PaLearn_VehiclePrm,RteInputBus.Reset.MtrCtrl_HIDO_SeatsButtonResetReq,LearnOut.MtrCtrl_LearnSts,RteInputBus.Reset.PaLearn_HeightAutoRunFlag,RteInputBus.Reset.PaLearn_LengthAutoRunFlag,RteInputBus.Reset.PaLearn_BackAutoRunFlag,RteInputBus.Reset.PaLearn_FrontAutoRunFlag,ResetReq,RteInputBus.Reset.MtrCtrl_BackGear_4Posi,RteInputBus.Reset.MtrCtrl_LengthGear_0Posi,RteInputBus.Reset.MtrCtrl_enFrontGear_0Posi,LearnCondition,RteInputBus.LearnDescConditions.PaLearn_CurrMotorCtrlType
  Reset : Stateflow chart  TreatAsAtomicUnit=on
  ResetOutBus : Outport
  wires:
  ResetInBus/1 -> Bus Selector/1
  Bus Creator/1 -> ResetOutBus/1  "ResetOutBus"
  Reset/2(HeightPosiReq) -> Bus Creator/1
  Reset/3(LengthPosiReq) -> Bus Creator/2
  Reset/4(BackPosiReq) -> Bus Creator/3
  Reset/5(FrontPosiReq) -> Bus Creator/4
  Bus Selector/1 -> Reset/1(MtrCtrl_BackDefaultStopPos)  "<PaLearn_BackDefaultStopPos>"
  Bus Selector/2 -> Reset/2(MtrCtrl_LengthDefaultStopPos)  "<PaLearn_LengthDefaultStopPos>"
  Bus Selector/3 -> Reset/3(MtrCtrl_FrontDefaulStoptPos)  "<PaLearn_FrontDefaulStoptPos>"
  Bus Selector/4 -> Reset/4(MtrCtrl_HeightDefaultStopPos)  "<PaLearn_HeightDefaultStopPos>"
  Bus Selector/5 -> Reset/5(MtrCtrl_VehiclePrm)  "<PaLearn_VehiclePrm>"
  Bus Selector/6 -> Reset/6(MtrCtrl_HIDO_SeatsButtonResetReq)  "<MtrCtrl_HIDO_SeatsButtonResetReq>"
  Bus Selector/7 -> Reset/7(MtrCtrl_LearnSts)  "<MtrCtrl_LearnSts>"
  Bus Selector/8 -> Reset/8(HeightAutoMotorRunFlag)  "<PaLearn_HeightAutoRunFlag>"
  Bus Selector/9 -> Reset/9(LengthAutoMotorRunFlag)  "<PaLearn_LengthAutoRunFlag>"
  Bus Selector/10 -> Reset/10(BackAutoMotorRunFlag)  "<PaLearn_BackAutoRunFlag>"
  Bus Selector/11 -> Reset/11(FrontAutoMotorRunFlag)  "<PaLearn_FrontAutoRunFlag>"
  Bus Selector/12 -> Reset/12(ResetReq)  "<ResetReq>"
  Bus Selector/13 -> Reset/13(MtrCtrl_BackGear_4Posi)  "<MtrCtrl_BackGear_4Posi>"
  Bus Selector/14 -> Reset/14(MtrCtrl_LengthGear_0Posi)  "<MtrCtrl_LengthGear_0Posi>"
  Bus Selector/15 -> Reset/15(MtrCtrl_enFrontGear_0Posi)  "<MtrCtrl_enFrontGear_0Posi>"
  Bus Selector/16 -> Reset/16(LearnCondition)  "<LearnCondition>"
  Bus Selector/17 -> Reset/17(MtrCtrl_CurrMotorCtrlType)  "<PaLearn_CurrMotorCtrlType>"

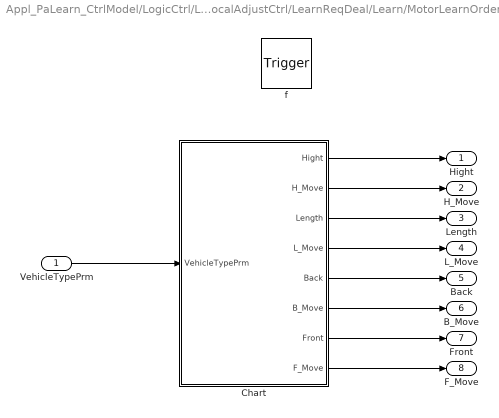
== system Appl_PaLearn_CtrlModel/LogicCtrl/LocalAdjustCtrl/LearnReqDeal/Learn/MotorLearnOrderPrm ==
  VehicleTypePrm : Inport
  f : TriggerPort  TriggerType=function-call  VariantControl=(inherit)
      settings: CopyFcn=Stateflow.SLINSF.SimulinkMan.removeBlockPreDeleteFcn  PreDeleteFcn=Stateflow.SLINSF.SimulinkMan.unsafePredeleteFcn
  Chart : Stateflow chart  TreatAsAtomicUnit=on
  Hight : Outport
  H_Move : Outport  Port=2
  Length : Outport  Port=3
  L_Move : Outport  Port=4
  Back : Outport  Port=5
  B_Move : Outport  Port=6
  Front : Outport  Port=7
  F_Move : Outport  Port=8
  wires:
  VehicleTypePrm/1 -> Chart/1(VehicleTypePrm)
  Chart/1(Hight) -> Hight/1
  Chart/2(H_Move) -> H_Move/1
  Chart/3(Length) -> Length/1
  Chart/4(L_Move) -> L_Move/1
  Chart/5(Back) -> Back/1
  Chart/6(B_Move) -> B_Move/1
  Chart/7(Front) -> Front/1
  Chart/8(F_Move) -> F_Move/1

== system Appl_PaLearn_CtrlModel/LogicCtrl/LocalAdjustCtrl/LearnReqDeal/Learn/SetDescLearnSts ==
  Sts : Inport
  f : TriggerPort  TriggerType=function-call  VariantControl=(inherit)
      settings: CopyFcn=Stateflow.SLINSF.SimulinkMan.removeBlockPreDeleteFcn  PreDeleteFcn=Stateflow.SLINSF.SimulinkMan.unsafePredeleteFcn
  setAPI_type3 : DareLib/Dare/setAPI_type  g_funcname=Rte_SetVfb_DrLearnEnable  g_param=""  g_type=uint8  g_size=-1
      settings: AttributesFormatString=%<g_funcname>  SourceProductName=Dare Library
  wires:
  Sts/1 -> setAPI_type3/1

== system Appl_PaLearn_CtrlModel/LogicCtrl/LocalAdjustCtrl/LearnReqDeal/Learn/SetDescLearnStsForDebug ==
  Sts : Inport
  f : TriggerPort  TriggerType=function-call  VariantControl=(inherit)
      settings: CopyFcn=Stateflow.SLINSF.SimulinkMan.removeBlockPreDeleteFcn  PreDeleteFcn=Stateflow.SLINSF.SimulinkMan.unsafePredeleteFcn
  setAPI_type3 : DareLib/Dare/setAPI_type  g_funcname=Srvl_Set_D_SimuIndex_DrLearnEnable  g_param=D_SimuIndex_DrLearnEnable  g_type=uint8  g_size=-1
      settings: AttributesFormatString=%<g_funcname>  SourceProductName=Dare Library
  wires:
  Sts/1 -> setAPI_type3/1

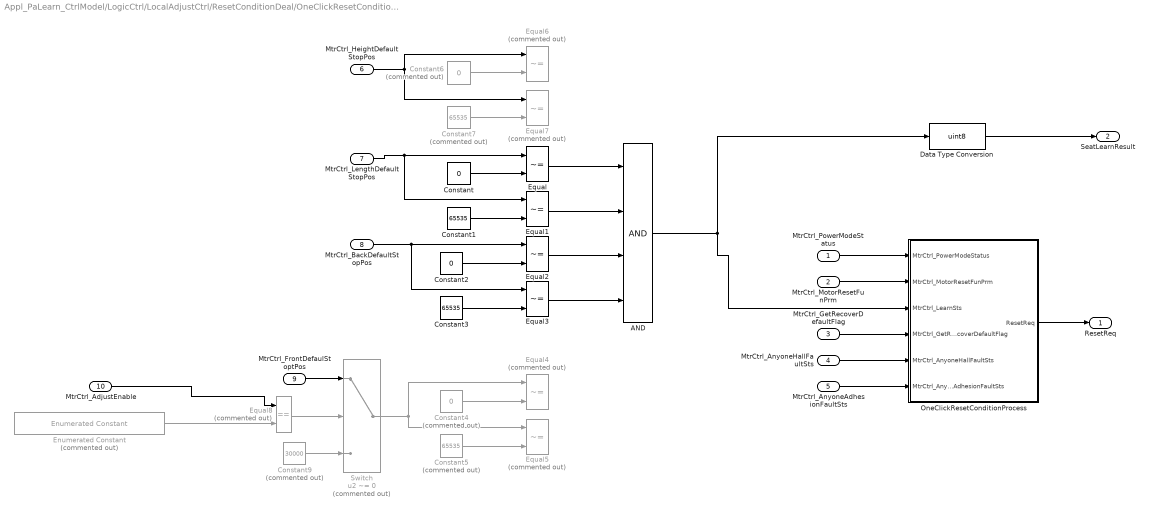
== system Appl_PaLearn_CtrlModel/LogicCtrl/LocalAdjustCtrl/ResetConditionDeal/OneClickResetConditionProcess ==
  MtrCtrl_PowerModeStatus : Inport
  MtrCtrl_MotorResetFunPrm : Inport  Port=2
  MtrCtrl_GetRecoverDefaultFlag : Inport  Port=3
  MtrCtrl_AnyoneHallFaultSts : Inport  Port=4
  MtrCtrl_AnyoneAdhesionFaultSts : Inport  Port=5
  MtrCtrl_HeightDefaultStopPos : Inport  Port=6
  MtrCtrl_LengthDefaultStopPos : Inport  Port=7
  MtrCtrl_BackDefaultStopPos : Inport  Port=8
  MtrCtrl_FrontDefaulStoptPos : Inport  Port=9
  MtrCtrl_AdjustEnable : Inport  Port=10
  AND : Logic  Inputs=4  AllPortsSameDT=off  OutDataTypeStr=boolean
  Constant : Constant  Value=0
  Constant1 : Constant  Value=65535
  Constant2 : Constant  Value=0
  Constant3 : Constant  Value=65535
  Constant4 : Constant  Commented=on  Value=0
  Constant5 : Constant  Commented=on  Value=65535
  Constant6 : Constant  Commented=on  Value=0
  Constant7 : Constant  Commented=on  Value=65535
  Constant9 : Constant  Commented=on  Value=30000
  Data Type Conversion : DataTypeConversion  OutDataTypeStr=uint8
  Enumerated Constant : simulink/Sources/Enumerated Constant  Commented=on  OutDataTypeStr=Enum: enDrAdjustEnable  Value=enDrAdjustEnable.EN_DrTwelveWayMotor  SampleTime=inf
      settings: SourceProductName=Simulink
  Equal{,1..3} (4 alike) : RelationalOperator  Operator=~=  OutDataTypeStr=boolean  RndMeth=Simplest
  Equal{4..7} (4 alike) : RelationalOperator  Commented=on  Operator=~=  OutDataTypeStr=boolean  RndMeth=Simplest
  Equal8 : RelationalOperator  Commented=on  Operator===  OutDataTypeStr=boolean  RndMeth=Simplest
  OneClickResetConditionProcess : Stateflow chart  TreatAsAtomicUnit=on
  Switch : Switch  Commented=on  Criteria=u2 ~= 0
  ResetReq : Outport
  SeatLearnResult : Outport  Port=2
  wires:
  MtrCtrl_AnyoneAdhesionFaultSts/1 -> OneClickResetConditionProcess/6(MtrCtrl_AnyoneAdhesionFaultSts)
  MtrCtrl_AnyoneHallFaultSts/1 -> OneClickResetConditionProcess/5(MtrCtrl_AnyoneHallFaultSts)
  OneClickResetConditionProcess/1(ResetReq) -> ResetReq/1
  MtrCtrl_PowerModeStatus/1 -> OneClickResetConditionProcess/1(MtrCtrl_PowerModeStatus)
  MtrCtrl_MotorResetFunPrm/1 -> OneClickResetConditionProcess/2(MtrCtrl_MotorResetFunPrm)
  AND/1 -> OneClickResetConditionProcess/3(MtrCtrl_LearnSts), Data Type Conversion/1
  MtrCtrl_GetRecoverDefaultFlag/1 -> OneClickResetConditionProcess/4(MtrCtrl_GetRecoverDefaultFlag)
  MtrCtrl_LengthDefaultStopPos/1 -> Equal1/1, Equal/1
  Constant/1 -> Equal/2
  Constant1/1 -> Equal1/2
  MtrCtrl_BackDefaultStopPos/1 -> Equal3/1, Equal2/1
  Constant2/1 -> Equal2/2
  Constant3/1 -> Equal3/2
  Constant5/1 -> Equal5/2
  Constant4/1 -> Equal4/2
  Constant7/1 -> Equal7/2
  Constant6/1 -> Equal6/2
  MtrCtrl_HeightDefaultStopPos/1 -> Equal6/1, Equal7/1
  Data Type Conversion/1 -> SeatLearnResult/1
  Enumerated Constant/1 -> Equal8/2
  MtrCtrl_AdjustEnable/1 -> Equal8/1
  Equal8/1 -> Switch/2
  MtrCtrl_FrontDefaulStoptPos/1 -> Switch/1
  Constant9/1 -> Switch/3
  Switch/1 -> Equal4/1, Equal5/1
  Equal/1 -> AND/1
  Equal1/1 -> AND/2
  Equal2/1 -> AND/3
  Equal3/1 -> AND/4

== stateflow chart Appl_PaLearn_CtrlModel/LogicCtrl/LocalAdjustCtrl/LearnConditionDeal/AutoLearnCmdProcess ==
  settings: description=自动学习调节命令处理
  note: /*公共前置条件判断
      |                                        D_RelayVolMinValue : 9V; D_RelayVolMaxValue:16V
      |                                        VoltFilterTime :200ms*/
  state PublicPreconditionJudgment
    state Enable/*条件满足*/
      en:
      LearnCondition = TRUE;
      LearnConditionExitCause  = enInvalid;
    state Disable/*条件不满足*/
      en:
      LearnCondition = FALSE;
    (default) -> Enable/*条件满足*
    Disable/*条件不满足* -> Enable/*条件满足* : /*电压在9-16V、非OTA
        | 无霍尔故障、继电器粘连故障、车速条件满足*/
        | [TRUE == VoltConditionSatisfy ...
        | && FALSE == MtrCtrl_OTAMode ...
        | &&FALSE == MtrCtrl_AnyoneHallFaultSts ...
        | &&FALSE == MtrCtrl_AnyoneAdhesionFaultSts ...
        | &&TRUE == MtrCtrl_VehSpdUnder3KMFlag ...
        | && EN_ManualEnable != MtrCtrl_CurrMotorCtrlType ...
        | && MtrCtrl_AdjustEnable != 0 ...
        | && MtrWel_WelcomeEnable != 0]
    Enable/*条件满足* -> Disable/*条件不满足* [order 1] : /*电压非9-16V、OTA
        | 任一霍尔故障、继电器粘连故障、车速条件不满足*/
        | [FALSE != MtrCtrl_AnyoneAdhesionFaultSts]
        | / LearnConditionExitCause  = enRelayAdhesionFault
    Enable/*条件满足* -> Disable/*条件不满足* [order 2] : [FALSE != MtrCtrl_AnyoneHallFaultSts]
        | /LearnConditionExitCause  =  enHallFault
    Enable/*条件满足* -> Disable/*条件不满足* [order 3] : [FALSE != MtrCtrl_OTAMode]
        | /LearnConditionExitCause  = enOTA
    Enable/*条件满足* -> Disable/*条件不满足* [order 4] : [TRUE != MtrCtrl_VehSpdUnder3KMFlag]
        | /LearnConditionExitCause  = enVehSpeed
    Enable/*条件满足* -> Disable/*条件不满足* [order 5] : [EN_ManualEnable ==MtrCtrl_CurrMotorCtrlType]
        | /LearnConditionExitCause  = enManualInterupt
    Enable/*条件满足* -> Disable/*条件不满足* [order 6] : [FALSE == VoltConditionSatisfy]
        | /LearnConditionExitCause  = enVoltFault
    Enable/*条件满足* -> Disable/*条件不满足* [commented out] : [hasChanged(MtrCtrl_DescSession)]
        | /LearnConditionExitCause  = enDescStop
    Enable/*条件满足* -> Disable/*条件不满足* [order 7] : [MtrCtrl_AdjustEnable  == 0]
        | /LearnConditionExitCause  = enCfgW_ADJUST
    Enable/*条件满足* -> Disable/*条件不满足* [order 8] : [0 == MtrWel_WelcomeEnable]
        | /LearnConditionExitCause  = enCfgW_MEMORY
  note: 自动学习调节命令处理
      | /*学习退出原因*/
      | enInvalid (无效)
      | enRelayAdhesionFault（继电器故障）
      | enHallFault（霍尔故障）
      | enOTA（OTA）
      | enVehSpeed（车速超过）
      | enManualInterupt（手动中断）
      | enVoltFault（电压故障）
      | enLearnOverTime(学习超时)
      | enMotorRunOverTiem(单个单机运行时间时)
      | enDescStop(诊断停止)
  (default) -> PublicPreconditionJudgment
  data: VoltConditionSatisfy input; MtrCtrl_OTAMode input; MtrCtrl_CurrMotorCtrlType input; MtrCtrl_AnyoneHallFaultSts input; MtrCtrl_AnyoneAdhesionFaultSts input; LearnCondition output uint8; LearnConditionExitCause output Enum: enLearnExitCause; FALSE parameter; TRUE parameter; MtrCtrl_VehSpdUnder3KMFlag input; MtrCtrl_DescSession input; MtrCtrl_AdjustEnable input; MtrWel_WelcomeEnable input

== stateflow chart Appl_PaLearn_CtrlModel/LogicCtrl/LocalAdjustCtrl/ResetReqDeal/Reset ==
  state ResetLogicalDeal
    state PositionTransform [parallel]
      settings: executionOrder=1
      state BM400
        (default) -> (junction 71)
        BM400 -> (junction 71)
        (junction 71) -> (junction 74) [order 1] : /*反馈位置坐标*/
            | [Back == CurrentResetSts]
        (junction 71) -> (junction 78) [order 2]
        (junction 74) -> (junction 83) : {BackPosiReq= MtrCtrl_BackDefaultStopPos+MtrCtrl_BackGear_4Posi;}
        (junction 78) -> (junction 84) [order 1] : [Length == CurrentResetSts]
        (junction 78) -> (junction 79) [order 2]
        (junction 84) -> (junction 86) : {LengthPosiReq= MtrCtrl_LengthDefaultStopPos+MtrCtrl_LengthGear_0Posi;}
        (junction 79) -> (junction 89) [order 1] : [Front == CurrentResetSts]
        (junction 79) -> (junction 88) [order 2]
        (junction 89) -> (junction 91) : {FrontPosiReq= MtrCtrl_FrontDefaulStoptPos+MtrCtrl_enFrontGear_0Posi}
        (junction 88) -> (junction 93) [order 1] : [Height == CurrentResetSts]
        (junction 88) -> (junction 80) [order 2]
        (junction 93) -> (junction 95) : {HeightPosiReq= 0x00;}
        (junction 95) -> (junction 80)
        (junction 91) -> (junction 95)
        (junction 86) -> (junction 91)
        (junction 83) -> (junction 86)
        (junction 80) -> (junction 81)
      state P20
        en:
        /*轨道长度 50% */
        LengthPosiReq= MtrCtrl_LengthDefaultStopPos+521;
        BackPosiReq= MtrCtrl_BackDefaultStopPos+2180;
      (default) -> (junction 65)
      (junction 65) -> (junction 68) [order 1] : [enVehTypePrm.enP20 == MtrCtrl_VehiclePrm]
      (junction 65) -> BM400 [order 2]
      (junction 68) -> P20
    state ResetPosition [parallel]
      settings: executionOrder=2
      state Init
        en:
        MotorResetSts = 0;
        ResetReqCall = FALSE;
        ResetResult  =  0;
        SendTimer = 0;
        (default) -> (junction 230)
        Init -> (junction 230) [order 1]
        (junction 230) -> (junction 236) [order 1] : [1 == ResetType]
        (junction 230) -> (junction 225) [order 2]
        (junction 236) -> (junction 231) : {ResetSts = enResetSts.enResetWaiting;}
        (junction 231) -> (junction 225)
        (junction 225) -> (junction 234)
      state HeightReset
        en:
        ResetReqCall =TRUE;
        HeightResetGear = 0;
        CurrentResetSts = Height;
      state BackReset
        en:
        ResetReqCall =TRUE;
        BackResetGear= enBackGear_4;
        CurrentResetSts = Back;
      state Reseting
        en:
        MotorResetSts += 1;
      state LengthReset
        en:
        ResetReqCall =TRUE;
        LengthResetGear = enLengthGear_0;
        CurrentResetSts = Length;
      state FrontReset
        en:
        ResetReqCall =TRUE;
        FrontResetGear = enFrontGear_0;
        CurrentResetSts = Front;
      (default) -> Init
      Init -> Reseting [order 1]
      Reseting -> HeightReset [order 3] : /*高度复位*/
          | [Height == MotorResetSts ]
      Reseting -> BackReset [order 1] : /*靠背复位*/
          | [Back == MotorResetSts]
      HeightReset -> Reseting : [enSeatAutoRunSts.EN_SEAT_SUCCESS == HeightAutoMotorRunFlag]
          | /ResetResult += Height;
      BackReset -> Reseting : [enSeatAutoRunSts.EN_SEAT_SUCCESS == BackAutoMotorRunFlag]
          | /ResetResult += Back;
      Reseting -> FrontReset [order 4] : /*腿托复位*/
          | [Front == MotorResetSts ]
      Reseting -> LengthReset [order 2] : /*纵向复位*/
          | [Length == MotorResetSts ]
      LengthReset -> Reseting : [enSeatAutoRunSts.EN_SEAT_SUCCESS == LengthAutoMotorRunFlag]
          | /ResetResult += Length;
      FrontReset -> Reseting : [enSeatAutoRunSts.EN_SEAT_SUCCESS == FrontAutoMotorRunFlag]
          | /ResetResult += Front;
    state WaitTimeSet [parallel]
      settings: executionOrder=3
      (default) -> (junction 205)
      WaitTimeSet -> (junction 205)
      (junction 205) -> (junction 210)
      (junction 210) -> (junction 212) [order 1] : /* 复位时间 */
          | [RestTimer <= 200]
      (junction 210) -> (junction 216) [order 2]
      (junction 212) -> (junction 214) : {RestTimer += 1;}
      (junction 214) -> (junction 216)
      (junction 216) -> (junction 219)
  state ResetInit
    en:
    ResetReqCall = FALSE;
    LengthResetGear = enLengthGear.enNULL ;
    FrontResetGear = enFrontGear.enNULL ;
    BackResetGear = enBackGear.enNULL ;
    CurrentResetSts  = 0x00;
    ResetResult  = 0x00;
    BackPosiReq = 0x00;
    LengthPosiReq = 0x00;
    FrontPosiReq = 0x00;
    HeightPosiReq= 0x00;
    MotorResetSts = 0;
    SendTimer = 0;
    RestTimer = 0;
    ex:
    SendTimer = 0;
    RestTimer = 0;
    (default) -> (junction 118)
    ResetInit -> (junction 118) [order 1]
    (junction 118) -> (junction 121) [order 1] : [enVehTypePrm.enBM400 == MtrCtrl_VehiclePrm]
    (junction 118) -> (junction 123) [order 2] : {
        | Height =D_Invalid;
        | Length =  D_FirstMove;
        | Back =  D_SecondMove;
        | Front = D_Invalid;
        | }
    (junction 121) -> (junction 125)
    (junction 125) -> (junction 123)
    (junction 123) -> (junction 128)
    (junction 128) -> (junction 153) [order 1] : [(ResetSts == enResetSts.enResetFail)...
        | ||(ResetSts == enResetSts.enResetSuccess)]
    (junction 153) -> (junction 156) [order 1] : [SendTimer >10]
    (junction 128) -> (junction 163) [order 2]
    (junction 153) -> (junction 160) [order 2] : {SendTimer++;}
    (junction 156) -> (junction 158) : {ResetSts = enResetSts.enInactive;
        | SendTimer = 0;}
    (junction 160) -> (junction 163)
    (junction 158) -> (junction 160)
    (junction 163) -> (junction 166)
  (default) -> ResetInit
  ResetInit -> ResetLogicalDeal [order 1] : /*（满足复位条件且收到复位信号）或（学习状态变为成功）*/
      | [(TRUE == ResetReq ...
      | &&hasChangedTo(MtrCtrl_HIDO_SeatsButtonResetReq,0x01)) ...
      | && enVehTypePrm.enBM400 == MtrCtrl_VehiclePrm]
      | /ResetType = 1;
      | Height =D_Invalid;
      | Length =  D_SecondMove;
      | Back =   D_FirstMove;
      | Front = D_ThirdlyMove;
      | ResetSts = enResetSts.enResetWaiting;
  ResetInit -> ResetLogicalDeal [order 2] : [hasChangedTo(MtrCtrl_LearnSts,enLearnAllSuccess)]
      | /ResetType = 2;
      | Height =D_Invalid;
      | Length =  D_FirstMove;
      | Back =  D_SecondMove;
      | Front = D_Invalid;
  ResetLogicalDeal -> ResetInit [order 1] : /*复位成功*/
      | [ResetResult == (Height+Length+Back+Front) &&(1 ==ResetType)]
      | /ResetSts = enResetSts.enResetSuccess;
  ResetLogicalDeal -> ResetInit [order 4] : /*通过学习完成后复位的方式触发不反馈成功*/
      | [ResetResult == (Height+Length+Back+Front) &&(2 ==ResetType)]
      | /ResetSts = enResetSts.enInactive;
  ResetLogicalDeal -> ResetInit [order 2] : /*退出复位或者任意方向复位失败*/
      | [(FALSE == ResetReq ...
      | ||enSeatAutoRunSts.EN_SEAT_FAIL == HeightAutoMotorRunFlag...
      | || enSeatAutoRunSts.EN_SEAT_FAIL == BackAutoMotorRunFlag...
      | || enSeatAutoRunSts.EN_SEAT_FAIL == LengthAutoMotorRunFlag...
      | || enSeatAutoRunSts.EN_SEAT_FAIL == FrontAutoMotorRunFlag...
      | || hasChanged(MtrCtrl_VehiclePrm))...
      | && 1 == ResetType]
      | /ResetSts = enResetSts.enResetFail;
  ResetLogicalDeal -> ResetInit [order 3] : /*通过学习完成后复位的方式触发不反馈失败  且调节类型非复位行为 */
      | [(enSeatAutoRunSts.EN_SEAT_FAIL == HeightAutoMotorRunFlag...
      | || enSeatAutoRunSts.EN_SEAT_FAIL == BackAutoMotorRunFlag...
      | || enSeatAutoRunSts.EN_SEAT_FAIL == LengthAutoMotorRunFlag...
      | || enSeatAutoRunSts.EN_SEAT_FAIL == FrontAutoMotorRunFlag...
      | || LearnCondition == FALSE ...
      | || (RestTimer > 2 && MtrCtrl_CurrMotorCtrlType != enSeatMotorRunTye.EN_ResetEnable) ...
      | || hasChanged(MtrCtrl_VehiclePrm))...
      | && 2 == ResetType]
      | /ResetSts = enResetSts.enInactive;
  data: MtrCtrl_BackDefaultStopPos input; MtrCtrl_LengthDefaultStopPos input; MtrCtrl_FrontDefaulStoptPos input; MtrCtrl_HeightDefaultStopPos input; MtrCtrl_VehiclePrm input; MtrCtrl_HIDO_SeatsButtonResetReq input; MtrCtrl_LearnSts input; HeightAutoMotorRunFlag input; LengthAutoMotorRunFlag input; BackAutoMotorRunFlag input; FrontAutoMotorRunFlag input; Height local uint8; Length local uint8; Back local uint8; Front local uint8; CurrentResetSts local uint8; ResetResult local uint8; ResetReqCall output uint8; MotorResetSts local uint8; TRUE parameter; FALSE parameter; ResetReq input; HeightPosiReq output uint16; LengthPosiReq output uint16; BackPosiReq output uint16; FrontPosiReq output uint16; ResetSts output Enum: enResetSts; HeightResetGear local uint8; LengthResetGear local Enum: enLengthGear; BackResetGear local Enum: enBackGear; FrontResetGear local Enum: enFrontGear; MtrCtrl_BackGear_4Posi input; MtrCtrl_LengthGear_0Posi input; MtrCtrl_enFrontGear_0Posi input; D_FirstMove parameter; D_FourthlyMove parameter; D_Invalid parameter; D_SecondMove parameter; D_ThirdlyMove parameter; ResetType local uint8; SendTimer local uint8; LearnCondition input; RestTimer local uint8; MtrCtrl_CurrMotorCtrlType input

== stateflow chart Appl_PaLearn_CtrlModel/LogicCtrl/LocalAdjustCtrl/ResetConditionDeal/OneClickResetConditionProcess/OneClickResetConditionProcess ==
  settings: description=自动学习调节命令处理
  note: 一键复位条件处理（BM400）
  state Active
    en:
    ResetReq = TRUE;
  state Inactive
    en:
    ResetReq = FALSE;
  (default) -> Inactive
  Inactive -> Active : /*电源模式为ON档
      | 无霍尔故障、无继电器粘连故障
      | 已学习成功
      | 配置有一键复位功能*/
      | [eOn == MtrCtrl_PowerModeStatus ...
      | &&FALSE == MtrCtrl_AnyoneHallFaultSts ...
      | &&FALSE == MtrCtrl_AnyoneAdhesionFaultSts ...
      | && TRUE == MtrCtrl_LearnSts ...
      | &&TRUE == MtrCtrl_MotorResetFunPrm]
  Active -> Inactive [order 1] : /*电源模式非ON档*/
      | [eOn != MtrCtrl_PowerModeStatus]
  Active -> Inactive [order 2] : /*任一无霍尔故障*/
      | [TRUE == MtrCtrl_AnyoneHallFaultSts]
  Active -> Inactive [order 3] : /*无继电器粘连故障*/
      | [ FALSE == MtrCtrl_AnyoneAdhesionFaultSts]
  Active -> Inactive [order 4] : /*未学习*/
      | [TRUE != MtrCtrl_LearnSts]
  Active -> Inactive [order 5] : /*恢复出厂*/
      | [TRUE == MtrCtrl_GetRecoverDefaultFlag]
  Active -> Inactive [order 6] : /*复位电机配置*/
      | [FALSE == MtrCtrl_MotorResetFunPrm]
  data: MtrCtrl_PowerModeStatus input; MtrCtrl_MotorResetFunPrm input; MtrCtrl_LearnSts input; MtrCtrl_GetRecoverDefaultFlag input; MtrCtrl_AnyoneHallFaultSts input; MtrCtrl_AnyoneAdhesionFaultSts input; FALSE parameter; TRUE parameter; ResetReq output uint8
